simulink model "Lab4_s"  (R2024a)
settings: Solver=VariableStepAuto  StartTime=0.0  StopTime=10.0  RelTol=1e-3
values from neighbouring files (symbols this model uses):
  A = [0, 1 ... (first row only)    [Lab4.m]
  ALPHA = inv(-(C-D*K)*inv((A-B*K))*B+D)    [Lab4.m]
  B = [0 ... (first row only)    [Lab4.m]
  C = [Kt, 0]    [Lab4.m]
  K = place(A,B,lambdaK)    [Lab4.m]
  L = place(A',C',lambdaL)'    [Lab4.m]
  x1 = 0.022    [Lab4.m]
settings Model: Creator=luigi  LastModifiedBy=luigi

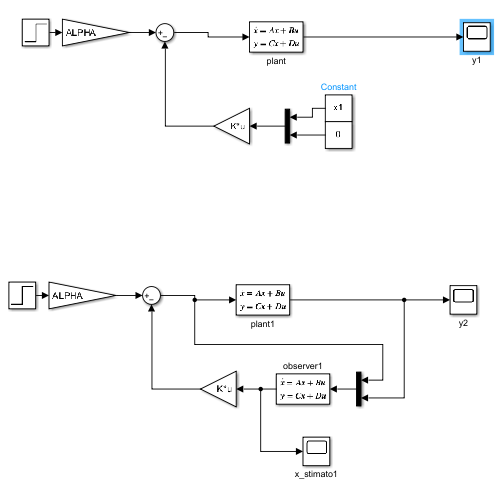
[thumbnail: Simulink's stored preview of the top-level diagram]
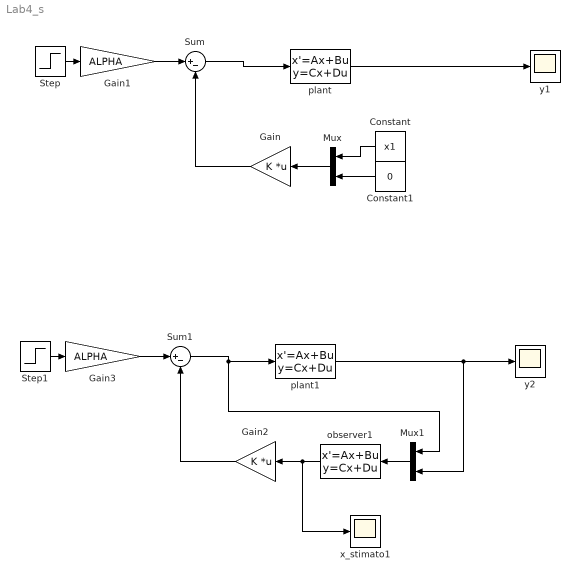
== system Lab4_s ==
  Constant : Constant  Value=x1
  Constant1 : Constant  Value=0
  Gain : Gain  Gain=K  Multiplication=Matrix(K*u)
  Gain1 : Gain  Gain=ALPHA
  Gain2 : Gain  Gain=K  Multiplication=Matrix(K*u)
  Gain3 : Gain  Gain=ALPHA
  Mux : Mux  Inputs=2
  Mux1 : Mux  Inputs=2
  Step : Step  Time=0  SampleTime=0
  Step1 : Step  Time=0  SampleTime=0
  Sum : Sum  Inputs=|+-
  Sum1 : Sum  Inputs=|+-
  observer1 : StateSpace  A=A-L*C  B="[B  L]"  C=eye(2)  D=zeros(2,2)  InitialCondition=[0 0]'
  plant : StateSpace  A=A  B=B  C=C  D=zeros(1,1)  InitialCondition=[0 0]'
  plant1 : StateSpace  A=A  B=B  C=C  D=0  InitialCondition=[0 0]'
  x_stimato1 : Scope
  y1 : Scope
  y2 : Scope
  wires:
  Gain/1 -> Sum/2
  plant/1 -> y1/1
  Gain1/1 -> Sum/1
  Sum/1 -> plant/1
  Step/1 -> Gain1/1
  Gain2/1 -> Sum1/2
  plant1/1 -> y2/1, Mux1/2
  Gain3/1 -> Sum1/1
  Sum1/1 -> Mux1/1, plant1/1
  observer1/1 -> x_stimato1/1, Gain2/1
  Mux1/1 -> observer1/1
  Step1/1 -> Gain3/1
  Mux/1 -> Gain/1
  Constant1/1 -> Mux/2
  Constant/1 -> Mux/1
